simulink model "act3_runge_kutta"  (R2021a)
settings: Solver=ode4  StartTime=0.0  StopTime=10.0  FixedStep=0.01  RelTol=1e-3
values from neighbouring files (symbols this model uses):
  a1 = 2    [exp1.m]    (also in main.m = 1)
  a2 = 1    [exp1.m]    (also in main.m = 2)
settings Model: Creator=zeta  LastModifiedBy=zeta

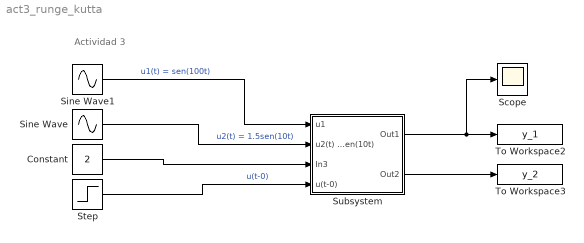
== system act3_runge_kutta ==
  note: Actividad 3
  Constant : Constant  Value=2
  Scope : Scope
  Sine Wave : Sin  Amplitude=1.5  Frequency=10  SampleTime=0
  Sine Wave1 : Sin  Frequency=100  SampleTime=0
  Step : Step  Time=0  SampleTime=0
  Subsystem : Subsystem
  To Workspace2 : ToWorkspace  VariableName=y_1  SampleTime=-1
  To Workspace3 : ToWorkspace  VariableName=y_2  SampleTime=-1
  wires:
  Subsystem/1(Out1) -> To Workspace2/1, Scope/1
  Sine Wave1/1 -> Subsystem/1(u1)  "u1(t) = sen(100t)"
  Sine Wave/1 -> Subsystem/2(u2(t) = 1.5sen(10t))  "u2(t) = 1.5sen(10t)"
  Constant/1 -> Subsystem/3(In3)
  Step/1 -> Subsystem/4(u(t-0))  "u(t-0)"
  Subsystem/2(Out2) -> To Workspace3/1

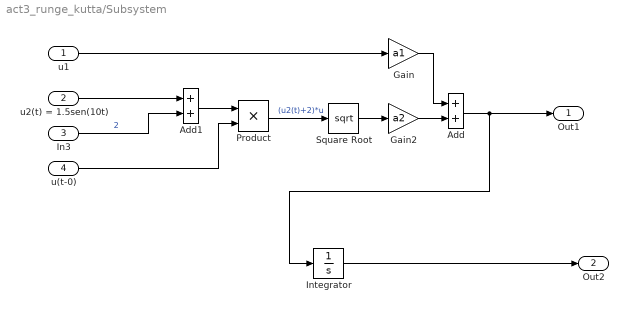
== system act3_runge_kutta/Subsystem ==
  u1 : Inport
  u2(t) = 1.5sen(10t) : Inport  Port=2
  In3 : Inport  Port=3
  u(t-0) : Inport  Port=4
  Add : Sum
  Add1 : Sum
  Gain : Gain  Gain=a1
  Gain2 : Gain  Gain=a2
  Integrator : Integrator
  Product : Product
  Square Root : Sqrt  SaturateOnIntegerOverflow=on
  Out1 : Outport
  Out2 : Outport  Port=2
  wires:
  u(t-0)/1 -> Product/2
  Add/1 -> Out1/1, Integrator/1
  Gain/1 -> Add/1
  Square Root/1 -> Gain2/1
  u1/1 -> Gain/1
  Product/1 -> Square Root/1  "(u2(t)+2)*u"
  u2(t) = 1.5sen(10t)/1 -> Add1/1
  Add1/1 -> Product/1
  Gain2/1 -> Add/2
  In3/1 -> Add1/2  "2"
  Integrator/1 -> Out2/1
